simulink model "bd_par_auto2"  (Simulink 4.1.1)
settings: Solver=ode1  SolverMode=SingleTasking  StartTime=0.0  StopTime=max(cyc_mph(:,1))  FixedStep=1  MaxStep=1  RelTol=1e-3  AbsTol=1e-3
undefined symbols (not defined in the file): air_cp, amb_tmp, cs_charge_deplete_bool, cs_charge_trq, cs_electric_decel_spd, cs_electric_launch_spd_hi, cs_electric_launch_spd_lo, cs_hi_soc, cs_lo_soc, cs_min_trq_frac, cs_off_trq_frac, cyc_avg_time, cyc_cargo_mass, cyc_elevation_init, cyc_filter_bool, cyc_grade, cyc_mph, enable_stop, ess_cap_scale, ess_coulombic_eff, ess_init_soc, ess_max_ah_cap, ess_max_volts, ess_min_volts, ess_mod_airflow, ess_mod_cp, ess_mod_init_tmp, ess_module_mass, ess_module_num, ess_on, ess_res_scale_coef, ess_res_scale_fun, ess_set_tmp, ess_th_calc, ess_th_res_off, ess_th_res_on, ess_tmp, ess_voc, ex_calc, fc_ct_trq, fc_emis, fc_inertia, fc_map_spd, fc_max_trq, fc_on, fc_spd_scale, fc_trq_scale, fc_tstat, fd_inertia, fd_loss, fd_ratio, gb_dnshift_load, gb_dnshift_spd, gb_gears_num, gb_inertia, gb_num_init, gb_ratio, gb_shift_delay, gb_spd_scale, gb_trq_scale ... (+56)
libraries: lib_wheel2 x12, lib_accessory2 x3, lib_etc x2, lib_drive_cycle2 x1, lib_interactive x1, lib_drive_cycle x1, lib_exhaust x1, lib_fuel_converter3 x1
(part 1 of 18)
settings Model: LastModifiedBy=mokeefe  ModifiedComment=mokeefe -- Wed Apr 16 13:36:53 2003 -- Version 1.22  SaveTime=off  SaveOutput=off  LimitDataPoints=off  UnconnectedLineMsg=none  RTWTemplateMakefile=grt_vc.tmf  ExtModeTrigMode=oneshot  ExtModeArmWhenConnect=off
settings Model: ModifiedHistory=|
  | mokeefe -- Wed Apr 16 13:36:53 2003 -- Version 1.22
  | 
  | 
  | mokeefe -- Wed Apr 16 13:36:31 2003 -- Version 1.21
  | 
  | 
  | mokeefe -- Fri Aug 30 07:45:49 2002 -- Version 1.20
  | Changed the input to "mechanical accessory loads <acc>/Mechanical Accessory Loads V2 <acc>" masked parameter input blocks. In R13, the function "not" no longer returns double 1 or double 0 for true and false but instead returns type logical (boolean). Thus, I am now multiplying by double 1 which causes a type conversion to double yielding the desired effect.
  | 
  | 
  | abrooker -- Tue May 14 11:45:21 2002 -- Version 1.19
  | 
  | 
  | mokeefe -- Thu Apr 18 08:00:10 2002 -- Version 1.18
  | saving the model:
  | o "without the model browser open"
  | o with only top-level screen visible
  | o and with "fit to view" enabled

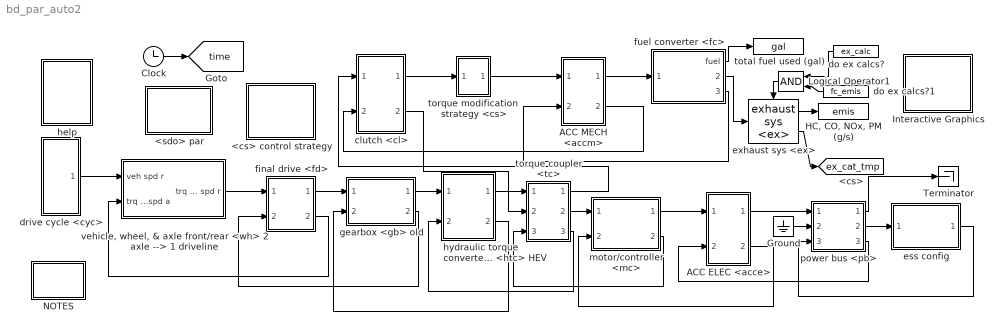
== system bd_par_auto2 ==
  <cs> control strategy : Subsystem
      settings: RTWFcnNameOpts=Auto  RTWFileNameOpts=Auto
      mask Display: image(imread('bdi_cs.jpg'))
  <sdo> par : Subsystem
      settings: RTWFcnNameOpts=Auto  RTWFileNameOpts=Auto
      mask Display: image(imread('bdi_sdo.jpg'))
  ACC ELEC <acce> : Subsystem  AncestorBlock=lib_accessory2/ACC ELEC <acce>  mask(Stand-Alone Electrical Accessory Mask){generalName='acce', logPick=Log, initFileName={}, modCell={}, imgFileName='bdi_acc_elec.bmp', DEBUG=OFF}
      mask prompts: generalName "General Name of this Component [char]"; logPick "Log Variables to Workspace?"; initFileName "Initialization File(s) [cell array of char]"; modCell "Modification Cell [2 column cell array of param and val]"; imgFileName "Icon image file name [char--evaluated]"
      mask init:
      | % initialization via m-file script
      | advSACompMaskInit;
      settings: RTWFcnNameOpts=Auto  RTWFileNameOpts=Auto
      mask StyleString: edit,popup(Don't Log|Log),edit,edit,edit,popup(ON|OFF)
      mask Display: image(imread(imgFileName))
  ACC MECH <accm> : Subsystem  AncestorBlock=lib_accessory2/ACC MECH <accm>  mask(Stand-Alone Mechanical Accessory Mask){generalName='accm', logPick=Log, initFileName={}, modCell={}, imgFileName='bdi_acc_pic.bmp', DEBUG=OFF}
      mask prompts: generalName "General Name of this Component [char]"; logPick "Log Variables to Workspace?"; initFileName "Initialization File(s) [cell array of char]"; modCell "Modification Cell [2 column cell array of param and val]"; imgFileName "Icon image file name [char--evaluated]"
      mask init:
      | % initialization via m-file script
      | advSACompMaskInit;
      settings: RTWFcnNameOpts=Auto  RTWFileNameOpts=Auto
      mask StyleString: edit,popup(Don't Log|Log),edit,edit,edit,popup(ON|OFF)
      mask Display: image(imread(imgFileName))
  Clock : Clock
      settings: DisplayTime=off  Decimation=10
  Ground : Ground
  "HC, CO, NOx, PM (g/s)" : ToWorkspace  VariableName=emis  SampleTime=0  SaveFormat=Array
  Interactive Graphics : Subsystem  BlockChoice=off
      settings: AttributesFormatString=%<BlockChoice>  TemplateBlock=lib_interactive/Interactive Graphics  MemberBlocks=off,on  RTWFcnNameOpts=Auto  RTWFileNameOpts=Auto
  Logical Operator1 : Logic  Orientation=left  Operator=AND  Inputs=2
  NOTES : Subsystem
      settings: RTWFcnNameOpts=Auto  RTWFileNameOpts=Auto
      mask Display: disp('Version &\nCopyright')
  Terminator : Terminator
  clutch <cl> : Subsystem  AncestorBlock=lib_transmission2/clutch <cl>  mask(Stand-Alone Clutch Mask){generalName='cl', logPick=Don't Log, initFileName={}, modCell={}, imgFileName='bdi_cl.jpg', slip_spd=vc_launch_spd, maxtrq=max(fc_max_trq)*fc_trq_scale, DEBUG=OFF}
      mask prompts: generalName "General Name of this Component [char--evaluated]"; logPick "Log Variables to Workspace?"; initFileName "Initialization File(s) [cell array of char]"; modCell "Modification Cell [2 column cell array of param and val]"; imgFileName "Icon image file name [char--evaluated]"; slip_spd "Input shaft speed when clutch slips (rad/s):"; maxtrq "Maximum torque clutch can transmit:"
      mask help: Clutch for use with ADVISOR 2
      mask init:
      | % initialization via m-file script
      | advSACompMaskInit;
      settings: RTWFcnNameOpts=Auto  RTWFileNameOpts=Auto
      mask Help:
      | First input is req'd clutch output torque and speed, muxed together.
      | Second input is clutch state, with 1 => disengaged, 2 => slipping, and 3=> engaged.
      | Third input is available clutch input torque and limited clutch input speed.
      | First output is req'd clutch input torque and speed, muxed together.
      | Second output is available clutch output torque and limited clutch output speed.
      | The logic implemented by this block is as follows:
      |           IF (clutch is disengaged) THEN (req'd input torque=0), (req'd input speed=req'd output speed (the engine control is responsible for computing correct engine spin-down speed)), (avail. output torque=0), (limited output speed=req'd output speed)
      |           IF (clutch is slipping) THEN (req'd input torque=req'd output torque), (req'd input speed=user-defined slip speed), (avail. output torque=avail. input torque), (limited output speed=req'd output speed)
      |           IF (clutch is engaged) THEN (req'd input torque=req'd output torque), (req'd input speed=req'd output speed), (avail. output torque=avail. input torque), (limited output speed=limited input speed)
      | 
      | The clutch will transmit no more than its maximum torque as driving or braking torque.
      mask StyleString: edit,popup(Don't Log|Log),edit,edit,edit,edit,edit,popup(ON|OFF)
      mask Display: image(imread(imgFileName))
  do ex calcs? : Constant  Orientation=left  Value=ex_calc
  do ex calcs?1 : Constant  Orientation=left  Value=fc_emis
  drive cycle <cyc> : Subsystem  AncestorBlock=lib_drive_cycle2/drive cycle <cyc>  mask(Stand-Alone Drive Cycle Mask){generalName='cyc', logPick=Log, initFileName={}, modCell={}, imgFileName='bdi_cyc.jpg', DEBUG=OFF, veh_mass=veh_mass}
      mask prompts: generalName "General Name of this Component [char]"; logPick "Log Variables to Workspace?"; initFileName "Initialization File(s) [cell array of char]"; modCell "Modification Cell [2 column cell array of param and val]"; imgFileName "Icon image file name [char--evaluated]"; veh_mass "Vehicle Mass (kg)"
      mask init:
      | % initialization via m-file script
      | advSACompMaskInit;
      settings: RTWFcnNameOpts=Auto  RTWFileNameOpts=Auto
      mask StyleString: edit,popup(Don't Log|Log),edit,edit,edit,popup(ON|OFF),edit
      mask Display: image(imread(imgFileName))
  ess config : Subsystem  BlockChoice=energy storage <ess>
      link override energy storage <ess>/controlTag: GotoTag=essControl
      link override energy storage <ess>/energy storage <ess>/Model/compute current/enhancedToWorkspace2/To Workspace: VariableName=ess_current  SampleTime=-1  SaveFormat=Array
      link override energy storage <ess>/energy storage <ess>/Model/enhancedToWorkspace/To Workspace: VariableName=ess_pwr_out_r  SampleTime=-1  SaveFormat=Array
      link override energy storage <ess>/energy storage <ess>/Model/enhancedToWorkspace1/To Workspace: VariableName=ess_pwr_loss_a  SampleTime=-1  SaveFormat=Array
      link override energy storage <ess>/energy storage <ess>/Model/enhancedToWorkspace2/To Workspace: VariableName=ess_mod_tmp  SampleTime=-1  SaveFormat=Array
      link override energy storage <ess>/energy storage <ess>/Model/enhancedToWorkspace3/To Workspace: VariableName=ess_air_tmp  SampleTime=-1  SaveFormat=Array
      link override energy storage <ess>/energy storage <ess>/Model/enhancedToWorkspace4/To Workspace: VariableName=ess_air_th_pwr  SampleTime=-1  SaveFormat=Array
      link override energy storage <ess>/energy storage <ess>/Model/enhancedToWorkspace5/To Workspace: VariableName=ess_pwr_out_a  SampleTime=-1  SaveFormat=Array
      link override energy storage <ess>/reqOutTag: GotoTag=essReqOut  TagVisibility=global
      link override energy storage <ess>/sensorsTag: GotoTag=essSensors  TagVisibility=global
      settings: AttributesFormatString=%<BlockChoice>  TemplateBlock=lib_energy_storage2/ess config  MemberBlocks="Ultracapacitor  System,energy storage <ess>,energy storage <ess> RC,energy storage <ess> nnet,energy storage <ess> Saber,energy storage <ess> fundamental model,energy storage <ess> optima fundamental model"  RTWFcnNameOpts=Auto  RTWFileNameOpts=Auto
  exhaust sys <ex> : lib_exhaust/exhaust sys <ex>
  final drive <fd> : Subsystem  AncestorBlock=lib_transmission2/final drive <fd>  mask(Stand-Alone Final Drive Mask){generalName='fd', logPick=Log, initFileName={}, modCell={}, imgFileName='bdi_fd.jpg', DEBUG=OFF}
      mask prompts: generalName "General Name of this Component [char]"; logPick "Log Variables to Workspace?"; initFileName "Initialization File(s) [cell array of char]"; modCell "Modification Cell [2 column cell array of param and val]"; imgFileName "Icon image file name [char--evaluated]"
      mask init:
      | % initialization via m-file script
      | advSACompMaskInit;
      settings: RTWFcnNameOpts=Auto  RTWFileNameOpts=Auto
      mask StyleString: edit,popup(Don't Log|Log),edit,edit,edit,popup(ON|OFF)
      mask Display: image(imread(imgFileName))
  fuel converter <fc> : Subsystem  AncestorBlock=lib_fuel_converter3/fuel converter <fc>  mask(Stand-Alone IC ENGINE Mask){generalName='fc', logPick=Log, initFileName={}, modCell={}, imgFileName='bdi_fc.jpg', DEBUG=OFF}
      mask prompts: generalName "General Name of this Component [char]"; logPick "Log Variables to Workspace?"; initFileName "Initialization File(s) [cell array of char]"; modCell "Modification Cell [2 column cell array of param and val]"; imgFileName "Icon image file name [char--evaluated]"
      mask init:
      | % initialization via m-file script
      | advSACompMaskInit;
      settings: RTWFcnNameOpts=Auto  RTWFileNameOpts=Auto
      mask StyleString: edit,popup(Don't Log|Log),edit,edit,edit,popup(ON|OFF)
      mask Display: image(imread(imgFileName))
  gearbox <gb> old : Subsystem  AncestorBlock=lib_transmission2/gearbox <gb> old  mask(Stand-Alone Gearbox Mask){generalName='gb', logPick=Log, initFileName={}, modCell={}, imgFileName='bdi_gb.jpg', DEBUG=OFF}
      mask prompts: generalName "General Name of this Component [char]"; logPick "Log Variables to Workspace?"; initFileName "Initialization File(s) [cell array of char]"; modCell "Modification Cell [2 column cell array of param and val]"; imgFileName "Icon image file name [char--evaluated]"
      mask init:
      | % initialization via m-file script
      | advSACompMaskInit;
      settings: RTWFcnNameOpts=Auto  RTWFileNameOpts=Auto
      mask StyleString: edit,popup(Don't Log|Log),edit,edit,edit,popup(ON|OFF)
      mask Display: image(imread(imgFileName))
  help : Subsystem
      settings: OpenFcn=web(['file:\\\' which('advisor_doc.htm')]);  RTWFcnNameOpts=Auto  RTWFileNameOpts=Auto
      mask Display: image(imread('doc_man.jpg'))
  hydraulic torque converter <htc> HEV : Subsystem  AncestorBlock=|  mask(Stand-Alone HTC Mask){generalName='htc', logPick=Log, initFileName={}, modCell={}, imgFileName='bdi_htc.jpg', DEBUG=OFF}
      | lib_transmission2/hydraulic
      | torque
      | converter <htc>
      | HEV
      mask prompts: generalName "General Name of this Component [char]"; logPick "Log Variables to Workspace?"; initFileName "Initialization File(s) [cell array of char]"; modCell "Modification Cell [2 column cell array of param and val]"; imgFileName "Icon image file name [char--evaluated]"
      mask init:
      | % initialization via m-file script
      | advSACompMaskInit;
      settings: RTWFcnNameOpts=Auto  RTWFileNameOpts=Auto
      mask StyleString: edit,popup(Don't Log|Log),edit,edit,edit,popup(ON|OFF)
      mask Display: image(imread(imgFileName))
  motor/controller <mc> : Subsystem  AncestorBlock=lib_electric_machine2/motor//controller <mc>  mask(Stand-Alone Motor/Controller Mask){generalName='mc', logPick=Log, initFileName={}, modCell={}, imgFileName='bdi_mc.jpg', DEBUG=OFF}
      mask prompts: generalName "General Name of this Component [char]"; logPick "Log Variables to Workspace?"; initFileName "Initialization File(s) [cell array of char]"; modCell "Modification Cell [2 column cell array of param and val]"; imgFileName "Icon image file name [char--evaluated]"
      mask init:
      | % initialization via m-file script
      | advSACompMaskInit;
      settings: RTWFcnNameOpts=Auto  RTWFileNameOpts=Auto
      mask StyleString: edit,popup(Don't Log|Log),edit,edit,edit,popup(ON|OFF)
      mask Display: image(imread(imgFileName))
  power bus <pb> : Subsystem  AncestorBlock=lib_power_bus2/power bus <pb>  mask(Stand-Alone Power Bus Mask){generalName='pb', logPick=Log, initFileName={}, modCell={}, imgFileName='bdi_pb.jpg', DEBUG=OFF}
      mask prompts: generalName "General Name of this Component [char]"; logPick "Log Variables to Workspace?"; initFileName "Initialization File(s) [cell array of char]"; modCell "Modification Cell [2 column cell array of param and val]"; imgFileName "Icon image file name [char--evaluated]"
      mask init:
      | % initialization via m-file script
      | advSACompMaskInit;
      settings: RTWFcnNameOpts=Auto  RTWFileNameOpts=Auto
      mask StyleString: edit,popup(Don't Log|Log),edit,edit,edit,popup(ON|OFF)
      mask Display: image(imread(imgFileName))
  torque coupler <tc> : Subsystem  AncestorBlock=lib_transmission2/torque coupler <tc>  mask(Stand-Alone Torque Coupler Mask){generalName='tc', logPick=Don't Log, initFileName={}, modCell={}, imgFileName='bdi_tc.jpg', DEBUG=OFF}
      mask prompts: generalName "General Name of this Component [char--evaluated]"; logPick "Log Variables to Workspace?"; initFileName "Initialization File(s) [cell array of char]"; modCell "Modification Cell [2 column cell array of param and val]"; imgFileName "Icon image file name [char--evaluated]"
      mask init:
      | % initialization via m-file script
      | advSACompMaskInit;
      settings: RTWFcnNameOpts=Auto  RTWFileNameOpts=Auto
      mask StyleString: edit,popup(Don't Log|Log),edit,edit,edit,popup(ON|OFF)
      mask Display: image(imread(imgFileName))
  torque modification  strategy <cs> : Subsystem  mask(Stand-Alone Torque Modification Strategy Mask){generalName='tm', logPick=Log, initFileName={}, modCell={}, imgFileName='bdi_hybrid_cntrl.jpg', DEBUG=OFF}
      mask prompts: generalName "General Name of this Component [char]"; logPick "Log Variables to Workspace?"; initFileName "Initialization File(s) [cell array of char]"; modCell "Modification Cell [2 column cell array of param and val]"; imgFileName "Icon image file name [char--evaluated]"
      mask init:
      | % initialization via m-file script
      | advSACompMaskInit;
      settings: RTWFcnNameOpts=Auto  RTWFileNameOpts=Auto
      mask StyleString: edit,popup(Don't Log|Log),edit,edit,edit,popup(ON|OFF)
      mask Display: image(imread(imgFileName))
  total fuel used (gal) : ToWorkspace  VariableName=gal  SampleTime=0  SaveFormat=Array
  "vehicle, wheel, & axle front/rear <wh> 2 axle --> 1 driveline" : Subsystem  AncestorBlock=|  mask(Stand-Alone Vehicle, Wheel, & Axle Mask){generalName='veh', generalName01='wh', logPick=Log, initFileName={}, modCell={}, imgFileName='bdi_wh&veh.jpg', DEBUG=OFF}
      | lib_wheel2/vehicle, wheel, & axle
      | front//rear <wh>
      | 2 axle --> 1 driveline
      mask prompts: generalName "General Name of Vehicle Component [char]"; generalName01 "General Name of Wheel Component [char]"; logPick "Log Variables to Workspace?"; initFileName "Initialization File(s) for VEH and WH [cell array of char]"; modCell "Modification Cell [2 column cell array of param and val]"; imgFileName "Icon image file name [char--evaluated]"
      mask init:
      | % initialization via m-file script
      | advSACompMaskInit;
      settings: RTWFcnNameOpts=Auto  RTWFileNameOpts=Auto
      mask StyleString: edit,edit,popup(Don't Log|Log),edit,edit,edit,popup(ON|OFF)
      mask Display: image(imread(imgFileName))
  tag scope: ex_cat_tmp=global, time=global
  wires:
  "vehicle, wheel, & axle front/rear <wh> 2 axle --> 1 driveline"/1(trq & spd r) -> final drive <fd>/1("torque and speed req'd at output side of final drive (Nm), (rad/s)")
  final drive <fd>/2("torque and speed avail. at output side of final drive (Nm), (rad/s)") -> "vehicle, wheel, & axle front/rear <wh> 2 axle --> 1 driveline"/2(trq & spd a)
  final drive <fd>/1("torque and speed req'd at input side of final drive (Nm), (rad/s)") -> gearbox <gb> old/1("torque and speed req'd at output side of gearbox (Nm), (rad/s)")
  drive cycle <cyc>/1(req'd vehicle speed (m/s)) -> "vehicle, wheel, & axle front/rear <wh> 2 axle --> 1 driveline"/1(veh spd r)
  clutch <cl>/1(T & w input request) -> torque modification  strategy <cs>/1("original torque and speed req'd (Nm), (rad/s)")
  fuel converter <fc>/2(engine out emissions) -> exhaust sys <ex>/1
  do ex calcs?/1 -> Logical Operator1/1
  fuel converter <fc>/1(fuel) -> total fuel used (gal)/1
  exhaust sys <ex>/1 -> "HC, CO, NOx, PM (g/s)"/1
  Logical Operator1/1 -> exhaust sys <ex>/Enable
  do ex calcs?1/1 -> Logical Operator1/2
  Clock/1 -> [time]
  gearbox <gb> old/2("torque and speed avail. at output side of gearbox (Nm), (rad/s)") -> final drive <fd>/2("torque and speed avail. at input side of final drive (Nm), (rad/s)")
  clutch <cl>/2(T & w output achieved) -> torque coupler <tc>/2("torque and speed avail. at main input (Nm), (rad/s)")
  torque coupler <tc>/1("torque and speed req'd at main input to torque coupler (Nm), (rad/s)") -> clutch <cl>/1(T & w output requested)
  motor/controller <mc>/2("trq and spd out achieved ") -> torque coupler <tc>/3("torque and speed avail. at motor input to tc (Nm), (rad/s)")
  Ground/1 -> power bus <pb>/2(power available from source one (W))
  power bus <pb>/2(power req'd from source two (W)) -> ess config/1(power req'd into bus (W))
  power bus <pb>/1(power req'd from source one (W)) -> Terminator/1
  ess config/1(power available to bus (W)) -> power bus <pb>/3(power available from source two (W))
  torque coupler <tc>/2("torque and speed req'd at motor input to torque coupler (Nm), (rad/s)") -> motor/controller <mc>/1(trq and spd out requested)
  gearbox <gb> old/1("torque and speed req'd at input side of gearbox (Nm), (rad/s)") -> hydraulic torque converter <htc> HEV/1(T & w output requested)
  hydraulic torque converter <htc> HEV/1(T & w input requested) -> torque coupler <tc>/1("torque and speed req'd at output side of torque coupler (Nm), (rad/s)")
  hydraulic torque converter <htc> HEV/2(T & w output available) -> gearbox <gb> old/2("torque and speed avail. at input side of gearbox (Nm), (rad/s)")
  torque coupler <tc>/3("torque and speed avail. at output side of torque coupler (Nm), (rad/s)") -> hydraulic torque converter <htc> HEV/2(T & w input available)
  exhaust sys <ex>/2 -> [ex_cat_tmp]
  motor/controller <mc>/1(electric power in  requested) -> ACC ELEC <acce>/1(elec pwr out r (W))
  ACC ELEC <acce>/1(elec pwr in r (W)) -> power bus <pb>/1(req'd power output (W))
  power bus <pb>/3(output power  available at bus) -> ACC ELEC <acce>/2(elec pwr in a (W))
  ACC ELEC <acce>/2(elec pwr out a (W)) -> motor/controller <mc>/2(electric power in achieved)
  torque modification  strategy <cs>/1("modified torque and speed req'd (Nm), (rad/s)") -> ACC MECH <accm>/1(trq and spd out requested)
  ACC MECH <accm>/1(trq and spd in  requested) -> fuel converter <fc>/1(trq and spd out requested)
  fuel converter <fc>/3(trq and spd out achieved) -> ACC MECH <accm>/2(trq and spd in achieved)
  ACC MECH <accm>/2("trq and spd out achieved ") -> clutch <cl>/2(T & w input achieved)

== system bd_par_auto2/<cs> control strategy ==
  Automatic Transmission  Control : Subsystem
      settings: RTWFcnNameOpts=Auto  RTWFileNameOpts=Auto
  Clutch Control : Subsystem
      settings: RTWFcnNameOpts=Auto  RTWFileNameOpts=Auto
  Drive Cycle : Subsystem
      settings: RTWFcnNameOpts=Auto  RTWFileNameOpts=Auto
  Electrical Accessories : Subsystem
      settings: RTWFcnNameOpts=Auto  RTWFileNameOpts=Auto
  Fuel Converter Control parallel hybrid  ic engine : Subsystem
      settings: RTWFcnNameOpts=Auto  RTWFileNameOpts=Auto
  Hybrid  Engine Torque Modification Strategy : Subsystem
      settings: RTWFcnNameOpts=Auto  RTWFileNameOpts=Auto
      mask Display: image(imread('bdi_hybrid_cntrl.jpg'))
  Mechanical Accessories : Subsystem
      settings: RTWFcnNameOpts=Auto  RTWFileNameOpts=Auto
  Motor Controller : Subsystem
      settings: RTWFcnNameOpts=Auto  RTWFileNameOpts=Auto
  Power Bus : Subsystem
      settings: RTWFcnNameOpts=Auto  RTWFileNameOpts=Auto
  Wheel Control : Subsystem
      settings: RTWFcnNameOpts=Auto  RTWFileNameOpts=Auto

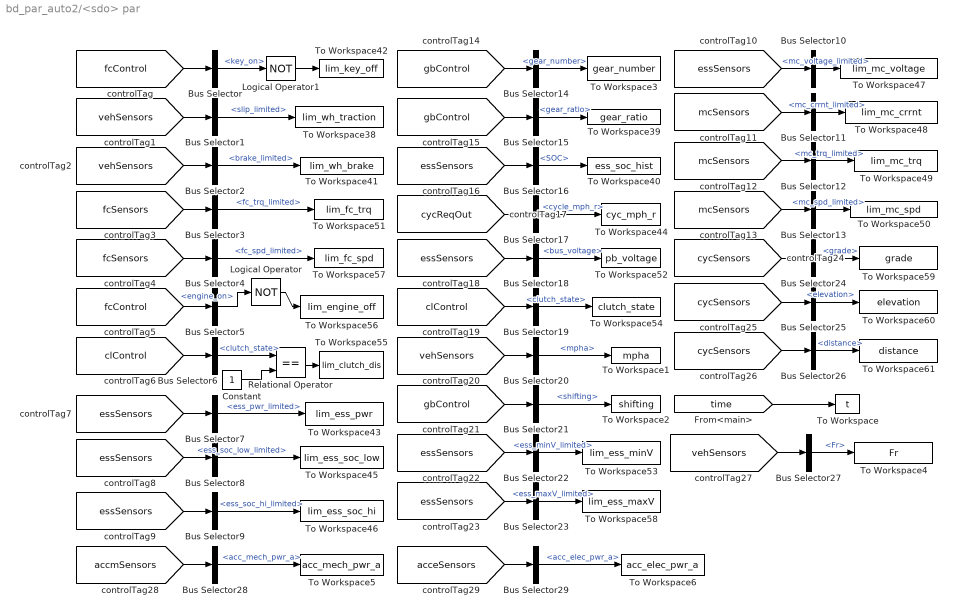
== system bd_par_auto2/<sdo> par ==
  Bus Selector : BusSelector  OutputSignals=key_on  MuxedOutput=off
  Bus Selector1 : BusSelector  OutputSignals=slip_limited  MuxedOutput=off
  Bus Selector10 : BusSelector  OutputSignals=mc_voltage_limited  MuxedOutput=off
  Bus Selector11 : BusSelector  OutputSignals=mc_crrnt_limited  MuxedOutput=off
  Bus Selector12 : BusSelector  OutputSignals=mc_trq_limited  MuxedOutput=off
  Bus Selector13 : BusSelector  OutputSignals=mc_spd_limited  MuxedOutput=off
  Bus Selector14 : BusSelector  OutputSignals=gear_number  MuxedOutput=off
  Bus Selector15 : BusSelector  OutputSignals=gear_ratio  MuxedOutput=off
  Bus Selector16 : BusSelector  OutputSignals=SOC  MuxedOutput=off
  Bus Selector17 : BusSelector  OutputSignals=cycle_mph_r  MuxedOutput=off
  Bus Selector18 : BusSelector  OutputSignals=bus_voltage  MuxedOutput=off
  Bus Selector19 : BusSelector  OutputSignals=clutch_state  MuxedOutput=off
  Bus Selector2 : BusSelector  OutputSignals=brake_limited  MuxedOutput=off
  Bus Selector20 : BusSelector  OutputSignals=mpha  MuxedOutput=off
  Bus Selector21 : BusSelector  OutputSignals=shifting  MuxedOutput=off
  Bus Selector22 : BusSelector  OutputSignals=ess_minV_limited  MuxedOutput=off
  Bus Selector23 : BusSelector  OutputSignals=ess_maxV_limited  MuxedOutput=off
  Bus Selector24 : BusSelector  OutputSignals=grade  MuxedOutput=off
  Bus Selector25 : BusSelector  OutputSignals=elevation  MuxedOutput=off
  Bus Selector26 : BusSelector  OutputSignals=distance  MuxedOutput=off
  Bus Selector27 : BusSelector  OutputSignals=Fr  MuxedOutput=off
  Bus Selector28 : BusSelector  OutputSignals=acc_mech_pwr_a  MuxedOutput=off
  Bus Selector29 : BusSelector  OutputSignals=acc_elec_pwr_a  MuxedOutput=off
  Bus Selector3 : BusSelector  OutputSignals=fc_trq_limited  MuxedOutput=off
  Bus Selector4 : BusSelector  OutputSignals=fc_spd_limited  MuxedOutput=off
  Bus Selector5 : BusSelector  OutputSignals=engine_on  MuxedOutput=off
  Bus Selector6 : BusSelector  OutputSignals=clutch_state  MuxedOutput=off
  Bus Selector7 : BusSelector  OutputSignals=ess_pwr_limited  MuxedOutput=off
  Bus Selector8 : BusSelector  OutputSignals=ess_soc_low_limited  MuxedOutput=off
  Bus Selector9 : BusSelector  OutputSignals=ess_soc_hi_limited  MuxedOutput=off
  Constant : Constant  Value=1
  Logical Operator : Logic  Operator=NOT  Inputs=1
  Logical Operator1 : Logic  Operator=NOT  Inputs=1
  Relational Operator : RelationalOperator  Operator===
  To Workspace : ToWorkspace  VariableName=t  SampleTime=0  SaveFormat=Array
  To Workspace1 : ToWorkspace  VariableName=mpha  SampleTime=-1  SaveFormat=Array
  To Workspace2 : ToWorkspace  VariableName=shifting  SampleTime=-1  SaveFormat=Array
  To Workspace3 : ToWorkspace  VariableName=gear_number  SampleTime=-1  SaveFormat=Array
  To Workspace38 : ToWorkspace  VariableName=lim_wh_traction  SampleTime=-1  SaveFormat=Array
  To Workspace39 : ToWorkspace  VariableName=gear_ratio  SampleTime=-1  SaveFormat=Array
  To Workspace4 : ToWorkspace  VariableName=Fr  SampleTime=-1  SaveFormat=Array
  To Workspace40 : ToWorkspace  VariableName=ess_soc_hist  SampleTime=-1  SaveFormat=Array
  To Workspace41 : ToWorkspace  VariableName=lim_wh_brake  SampleTime=-1  SaveFormat=Array
  To Workspace42 : ToWorkspace  VariableName=lim_key_off  SampleTime=-1  SaveFormat=Array
  To Workspace43 : ToWorkspace  VariableName=lim_ess_pwr  SampleTime=-1  SaveFormat=Array
  To Workspace44 : ToWorkspace  VariableName=cyc_mph_r  SampleTime=-1  SaveFormat=Array
  To Workspace45 : ToWorkspace  VariableName=lim_ess_soc_low  SampleTime=-1  SaveFormat=Array
  To Workspace46 : ToWorkspace  VariableName=lim_ess_soc_hi  SampleTime=-1  SaveFormat=Array
  To Workspace47 : ToWorkspace  VariableName=lim_mc_voltage  SampleTime=-1  SaveFormat=Array
  To Workspace48 : ToWorkspace  VariableName=lim_mc_crrnt  SampleTime=-1  SaveFormat=Array
  To Workspace49 : ToWorkspace  VariableName=lim_mc_trq  SampleTime=-1  SaveFormat=Array
  To Workspace5 : ToWorkspace  VariableName=acc_mech_pwr_a  SampleTime=-1  SaveFormat=Array
  To Workspace50 : ToWorkspace  VariableName=lim_mc_spd  SampleTime=-1  SaveFormat=Array
  To Workspace51 : ToWorkspace  VariableName=lim_fc_trq  SampleTime=-1  SaveFormat=Array
  To Workspace52 : ToWorkspace  VariableName=pb_voltage  SampleTime=-1  SaveFormat=Array
  To Workspace53 : ToWorkspace  VariableName=lim_ess_minV  SampleTime=-1  SaveFormat=Array
  To Workspace54 : ToWorkspace  VariableName=clutch_state  SampleTime=-1  SaveFormat=Array
  To Workspace55 : ToWorkspace  VariableName=lim_clutch_dis  SampleTime=-1  SaveFormat=Array
  To Workspace56 : ToWorkspace  VariableName=lim_engine_off  SampleTime=-1  SaveFormat=Array
  To Workspace57 : ToWorkspace  VariableName=lim_fc_spd  SampleTime=-1  SaveFormat=Array
  To Workspace58 : ToWorkspace  VariableName=lim_ess_maxV  SampleTime=-1  SaveFormat=Array
  To Workspace59 : ToWorkspace  VariableName=grade  SampleTime=-1  SaveFormat=Array
  To Workspace6 : ToWorkspace  VariableName=acc_elec_pwr_a  SampleTime=-1  SaveFormat=Array
  To Workspace60 : ToWorkspace  VariableName=elevation  SampleTime=-1  SaveFormat=Array
  To Workspace61 : ToWorkspace  VariableName=distance  SampleTime=-1  SaveFormat=Array
  wires:
  [time] -> To Workspace/1
  Logical Operator/1 -> To Workspace56/1
  Bus Selector1/1 -> To Workspace38/1  "<slip_limited>"
  Logical Operator1/1 -> To Workspace42/1
  [fcControl] -> Bus Selector/1
  Bus Selector/1 -> Logical Operator1/1  "<key_on>"
  [vehSensors] -> Bus Selector1/1
  Bus Selector2/1 -> To Workspace41/1  "<brake_limited>"
  [vehSensors] -> Bus Selector2/1
  [fcSensors] -> Bus Selector3/1
  Bus Selector3/1 -> To Workspace51/1  "<fc_trq_limited>"
  [fcSensors] -> Bus Selector4/1
  Bus Selector4/1 -> To Workspace57/1  "<fc_spd_limited>"
  [fcControl] -> Bus Selector5/1
  Bus Selector5/1 -> Logical Operator/1  "<engine_on>"
  [clControl] -> Bus Selector6/1
  Relational Operator/1 -> To Workspace55/1
  Constant/1 -> Relational Operator/2
  Bus Selector6/1 -> Relational Operator/1  "<clutch_state>"
  [essSensors] -> Bus Selector7/1
  Bus Selector7/1 -> To Workspace43/1  "<ess_pwr_limited>"
  [essSensors] -> Bus Selector8/1
  Bus Selector8/1 -> To Workspace45/1  "<ess_soc_low_limited>"
  [essSensors] -> Bus Selector9/1
  Bus Selector9/1 -> To Workspace46/1  "<ess_soc_hi_limited>"
  [essSensors] -> Bus Selector10/1
  Bus Selector10/1 -> To Workspace47/1  "<mc_voltage_limited>"
  [mcSensors] -> Bus Selector11/1
  Bus Selector11/1 -> To Workspace48/1  "<mc_crrnt_limited>"
  [mcSensors] -> Bus Selector12/1
  Bus Selector12/1 -> To Workspace49/1  "<mc_trq_limited>"
  [mcSensors] -> Bus Selector13/1
  Bus Selector13/1 -> To Workspace50/1  "<mc_spd_limited>"
  [gbControl] -> Bus Selector14/1
  Bus Selector14/1 -> To Workspace3/1  "<gear_number>"
  [gbControl] -> Bus Selector15/1
  Bus Selector15/1 -> To Workspace39/1  "<gear_ratio>"
  [essSensors] -> Bus Selector16/1
  Bus Selector16/1 -> To Workspace40/1  "<SOC>"
  [cycReqOut] -> Bus Selector17/1
  Bus Selector17/1 -> To Workspace44/1  "<cycle_mph_r>"
  [essSensors] -> Bus Selector18/1
  Bus Selector18/1 -> To Workspace52/1  "<bus_voltage>"
  [clControl] -> Bus Selector19/1
  Bus Selector19/1 -> To Workspace54/1  "<clutch_state>"
  [vehSensors] -> Bus Selector20/1
  Bus Selector20/1 -> To Workspace1/1  "<mpha>"
  [gbControl] -> Bus Selector21/1
  Bus Selector21/1 -> To Workspace2/1  "<shifting>"
  [essSensors] -> Bus Selector22/1
  Bus Selector22/1 -> To Workspace53/1  "<ess_minV_limited>"
  [essSensors] -> Bus Selector23/1
  Bus Selector23/1 -> To Workspace58/1  "<ess_maxV_limited>"
  [cycSensors] -> Bus Selector24/1
  Bus Selector24/1 -> To Workspace59/1  "<grade>"
  [cycSensors] -> Bus Selector25/1
  Bus Selector25/1 -> To Workspace60/1  "<elevation>"
  [cycSensors] -> Bus Selector26/1
  Bus Selector26/1 -> To Workspace61/1  "<distance>"
  [vehSensors] -> Bus Selector27/1
  Bus Selector27/1 -> To Workspace4/1  "<Fr>"
  [accmSensors] -> Bus Selector28/1
  Bus Selector28/1 -> To Workspace5/1  "<acc_mech_pwr_a>"
  [acceSensors] -> Bus Selector29/1
  Bus Selector29/1 -> To Workspace6/1  "<acc_elec_pwr_a>"

== system bd_par_auto2/ACC ELEC <acce> ==
  note: ELECTRICAL ACCESSORY
      | Interface
  elec pwr out r (W) : Inport  Port=1  LatchInput=off
  elec pwr in a (W) : Inport  Port=2  LatchInput=off
  ACC ELEC model and interface : lib_accessory2/ACC ELEC <acce>/ACC ELEC model and interface
      link override electrical accessory model/backward model/electrical accessories (W): BlockChoice=Electrical Accessories: Time Variable
  elec pwr in r (W) : Outport  Port=1
  elec pwr out a (W) : Outport  Port=2
  tag scope: acceReqOut=global, acceSensors=global
  wires:
  [acceControl] -> ACC ELEC model and interface/3
  elec pwr out r (W)/1 -> ACC ELEC model and interface/1
  elec pwr in a (W)/1 -> ACC ELEC model and interface/2
  ACC ELEC model and interface/1 -> [acceReqOut]
  ACC ELEC model and interface/2 -> elec pwr in r (W)/1
  ACC ELEC model and interface/3 -> elec pwr out a (W)/1
  ACC ELEC model and interface/4 -> [acceSensors]

== system bd_par_auto2/ACC MECH <accm> ==
  note: MECHANICAL ACCESSORY
      | Interface
  trq and spd out requested : Inport  Port=1  LatchInput=off
  trq and spd in achieved : Inport  Port=2  LatchInput=off
  mechanical accessory model and interface : Subsystem  AncestorBlock=lib_accessory2/ACC MECH <accm>/mechanical accessory model and interface
      settings: RTWFcnNameOpts=Auto  RTWFileNameOpts=Auto
  trq and spd in  requested : Outport  Port=1
  "trq and spd out achieved " : Outport  Port=2
  tag scope: accmReqOut=global, accmSensors=global
  wires:
  mechanical accessory model and interface/4(sensors) -> [accmSensors]
  [accmControl] -> mechanical accessory model and interface/3(control)
  mechanical accessory model and interface/1(Out Request) -> [accmReqOut]
  mechanical accessory model and interface/2(T,w in request) -> trq and spd in  requested/1
  trq and spd out requested/1 -> mechanical accessory model and interface/1("T, w out requested")
  trq and spd in achieved/1 -> mechanical accessory model and interface/2("T, w in achieved")
  mechanical accessory model and interface/3("T, w out achieved") -> "trq and spd out achieved "/1

== system bd_par_auto2/Interactive Graphics ==
  off : lib_interactive/off  Tag=Altia_off  Orientation=up

== system bd_par_auto2/NOTES ==
  note: ADVISOR software developed at NREL.  Copyright 1998 Midwest Research Institute.  All rights reserved.
      | Notice: These data were produced by the Midwest Research Institute (MRI) under Contract No. DE-AC98GO10337
      |      with the Department of Energy (DOE).  For a five-year period from November 6, 1998, the Government is granted for
      | itself and others acting on its behalf a nonexclusive, paid-up, irrevocable worldwide license in this data to reproduce,
      |  prepare derivative works, and perform publicly and display publicly, by or on behalf of the Government.  There is
      | provision for the possible extension of the term of this license.  Subsequent to that period or any extension granted,
      |  the Government is granted for itself and others acting on its behalf a nonexclusive, paid-up, irrevocable worldwide
  note: license in this data to reproduce, prepare derivative works, distribute copies to the public, perform publicly and display
      | publicly, and to permit others to do so.  The specific term of the license can be identified by inquiry made to the MRI
      | or DOE. Neither the United States nor the DOE, nor any of their employees, make any warranty, express or implied, or
      | assumes any legal liability or responsibility for the accuracy, completeness, or usefulness of any data, apparatus,
      | product, or process disclosed, or represents that its use would not infringe privately owned rights.
  NOTES : Subsystem
      settings: OpenFcn=advisor_ver  RTWFcnNameOpts=Auto  RTWFileNameOpts=Auto
      mask Display: disp('Double-click here or enter ''advisor_ver'' at the Matlab\ncommand line for ADVISOR version')

== system bd_par_auto2/clutch <cl> ==
  note: Clutch
      | Interface
  T & w output requested : Inport  Port=1  LatchInput=off
  T & w input achieved : Inport  Port=2  LatchInput=off
  clutch model and interface : Subsystem
      settings: RTWFcnNameOpts=Auto  RTWFileNameOpts=Auto
  T & w input request : Outport  Port=1
  T & w output achieved : Outport  Port=2
  tag scope: clReqOut=global, clSensors=global
  wires:
  [clControl] -> clutch model and interface/3(control)
  clutch model and interface/1(required out) -> [clReqOut]
  clutch model and interface/4(sensors) -> [clSensors]
  clutch model and interface/3(Out2) -> T & w output achieved/1
  T & w input achieved/1 -> clutch model and interface/2(T & w input achieved)
  clutch model and interface/2(Out1) -> T & w input request/1
  T & w output requested/1 -> clutch model and interface/1(T & w output requested)

== system bd_par_auto2/drive cycle <cyc> ==
  note: DRIVE CYCLE
  drive cycle model and interface : Subsystem
      settings: RTWFcnNameOpts=Auto  RTWFileNameOpts=Auto
  req'd vehicle speed (m/s) : Outport  Port=1  InitialOutput=0
  tag scope: cycReqOut=global, cycSensors=global
  wires:
  drive cycle model and interface/3(sensors) -> [cycSensors]
  drive cycle model and interface/1(req'd lookups) -> [cycReqOut]
  [cycControl] -> drive cycle model and interface/1(control)
  drive cycle model and interface/2(req'd vehicle speed (m/s)) -> req'd vehicle speed (m/s)/1

== system bd_par_auto2/ess config ==
  power req'd into bus (W) : Inport  Port=1  LatchInput=off
  energy storage <ess> : Subsystem  AncestorBlock=lib_energy_storage2/energy storage <ess>  mask(Stand-Alone Energy Storage System Mask){generalName='ess', logPick=Log Variable, initFileName={}, modCell={}, imgFileName='bdi_ess.jpg', DEBUG=OFF}
      mask prompts: generalName "General Name of this Component [char]"; logPick "Log Variables to Workspace?"; initFileName "Initialization File(s) [cell array of char]"; modCell "Modification Cell [2 column cell array of param and val]"; imgFileName "Icon image file name [char--evaluated]"
      mask init:
      | % initialization via m-file script
      | advSACompMaskInit;
      settings: RTWFcnNameOpts=Auto  RTWFileNameOpts=Auto
      mask StyleString: edit,popup(Don't Log|Log Variable),edit,edit,edit,popup(ON|OFF)
      mask Display: image(imread(imgFileName))
  power available to bus (W) : Outport  Port=1
  wires:
  power req'd into bus (W)/1 -> energy storage <ess>/1(power req'd into bus (W))
  energy storage <ess>/1(power available to bus (W)) -> power available to bus (W)/1

== system bd_par_auto2/final drive <fd> ==
  "torque and speed req'd at output side of final drive (Nm), (rad/s)" : Inport  Port=1  LatchInput=off
  "torque and speed avail. at input side of final drive (Nm), (rad/s)" : Inport  Port=2  LatchInput=off
  Block NOTES : Subsystem
      settings: RTWFcnNameOpts=Auto  RTWFileNameOpts=Auto
      mask Display: disp('Block\nNOTES')
  help : Subsystem
      settings: OpenFcn=web(['file:\\\' which('wheel_axle.htm')]);  RTWFcnNameOpts=Auto  RTWFileNameOpts=Auto
      mask Display: image(imread('doc_man.jpg'))
  model&interface : Subsystem
      settings: RTWFcnNameOpts=Auto  RTWFileNameOpts=Auto
  "torque and speed req'd at input side of final drive (Nm), (rad/s)" : Outport  Port=1  InitialOutput=0
  "torque and speed avail. at output side of final drive (Nm), (rad/s)" : Outport  Port=2  InitialOutput=0
  tag scope: fdReqOut=global, fdSensors=global
  wires:
  model&interface/3(T & w output achieved) -> "torque and speed avail. at output side of final drive (Nm), (rad/s)"/1
  model&interface/2(T & w input request) -> "torque and speed req'd at input side of final drive (Nm), (rad/s)"/1
  "torque and speed avail. at input side of final drive (Nm), (rad/s)"/1 -> model&interface/2(T & w input achieved)
  "torque and speed req'd at output side of final drive (Nm), (rad/s)"/1 -> model&interface/1(T & w output request)
  model&interface/4(sensors) -> [fdSensors]
  [fdControl] -> model&interface/3(control)
  model&interface/1(out request) -> [fdReqOut]

== system bd_par_auto2/fuel converter <fc> ==
  note: Internal Combustion Engine
  trq and spd out requested : Inport  Port=1  LatchInput=off
  Block NOTES : Subsystem
      settings: RTWFcnNameOpts=Auto  RTWFileNameOpts=Auto
      mask Display: disp('Block\nNOTES')
  IC Engine Model  &  Interface : Subsystem
      settings: RTWFcnNameOpts=Auto  RTWFileNameOpts=Auto
  help : Subsystem
      settings: OpenFcn=web(['file:\\\' which('fuel_converter.htm')]);  RTWFcnNameOpts=Auto  RTWFileNameOpts=Auto
      mask Display: image(imread('doc_man.jpg'))
  fuel : Outport  Port=1
  engine out emissions : Outport  Port=2
  trq and spd out achieved : Outport  Port=3
  tag scope: fcReqOut=global, fcSensors=global
  wires:
  IC Engine Model  &  Interface/1(req out) -> [fcReqOut]
  IC Engine Model  &  Interface/2(fuel) -> fuel/1
  IC Engine Model  &  Interface/3(engine out emissions) -> engine out emissions/1
  IC Engine Model  &  Interface/4(trq and spd out achieved) -> trq and spd out achieved/1
  IC Engine Model  &  Interface/5(sensors) -> [fcSensors]
  [fcControl] -> IC Engine Model  &  Interface/2(control)
  trq and spd out requested/1 -> IC Engine Model  &  Interface/1(trq and spd out requested)

== system bd_par_auto2/gearbox <gb> old ==
  note: Gearbox
  "torque and speed req'd at output side of gearbox (Nm), (rad/s)" : Inport  Port=1  LatchInput=off
  "torque and speed avail. at input side of gearbox (Nm), (rad/s)" : Inport  Port=2  LatchInput=off
  Block NOTES : Subsystem
      settings: RTWFcnNameOpts=Auto  RTWFileNameOpts=Auto
      mask Display: disp('Block\nNOTES')
  gearbox model & interface : Subsystem
      settings: RTWFcnNameOpts=Auto  RTWFileNameOpts=Auto
  help : Subsystem
      settings: OpenFcn=web(['file:\\\' which('gearbox.htm')]);  RTWFcnNameOpts=Auto  RTWFileNameOpts=Auto
      mask Display: image(imread('doc_man.jpg'))
  "torque and speed req'd at input side of gearbox (Nm), (rad/s)" : Outport  Port=1  InitialOutput=0
  "torque and speed avail. at output side of gearbox (Nm), (rad/s)" : Outport  Port=2  InitialOutput=0
  tag scope: gbReqOut=global, gbSensors=global
  wires:
  gearbox model & interface/4(sensors) -> [gbSensors]
  [gbControl] -> gearbox model & interface/3(controls)
  gearbox model & interface/3(trq and spd output achieved) -> "torque and speed avail. at output side of gearbox (Nm), (rad/s)"/1
  "torque and speed avail. at input side of gearbox (Nm), (rad/s)"/1 -> gearbox model & interface/2(trq and spd input achieved)
  "torque and speed req'd at output side of gearbox (Nm), (rad/s)"/1 -> gearbox model & interface/1(trq and spd output request)
  gearbox model & interface/2(trq and spd input request) -> "torque and speed req'd at input side of gearbox (Nm), (rad/s)"/1
  gearbox model & interface/1(requested output) -> [gbReqOut]

== system bd_par_auto2/help ==

== system bd_par_auto2/hydraulic torque converter <htc> HEV ==
  note: Hydraulic Torque Converter
  T & w output requested : Inport  Port=1  LatchInput=off
  T & w input available : Inport  Port=2  LatchInput=off
  HTC for parallel HEV and Interface : Subsystem
      settings: RTWFcnNameOpts=Auto  RTWFileNameOpts=Auto
  T & w input requested : Outport  Port=1  InitialOutput=0
  T & w output available : Outport  Port=2  InitialOutput=0
  tag scope: htcReqOut=global, htcSensors=global
  wires:
  [htcControl] -> HTC for parallel HEV and Interface/3(control)
  T & w input available/1 -> HTC for parallel HEV and Interface/2(trq and spd input achieved)
  T & w output requested/1 -> HTC for parallel HEV and Interface/1(trq and spd output request)
  HTC for parallel HEV and Interface/3(trq and spd output achieved) -> T & w output available/1
  HTC for parallel HEV and Interface/2(trq and spd input request) -> T & w input requested/1
  HTC for parallel HEV and Interface/4(sensors) -> [htcSensors]
  HTC for parallel HEV and Interface/1(requested output) -> [htcReqOut]

== system bd_par_auto2/motor/controller <mc> ==
  note: MOTOR/ CONTROLLER
      | Interface
  trq and spd out requested : Inport  Port=1  LatchInput=off
  electric power in achieved : Inport  Port=2  LatchInput=off
  motor model & interface : Subsystem
      settings: RTWFcnNameOpts=Auto  RTWFileNameOpts=Auto
  electric power in  requested : Outport  Port=1
  "trq and spd out achieved " : Outport  Port=2
  tag scope: mcReqOut=global, mcSensors=global
  wires:
  motor model & interface/3("trq and spd out achieved ") -> "trq and spd out achieved "/1
  electric power in achieved/1 -> motor model & interface/2(electric power in achieved)
  trq and spd out requested/1 -> motor model & interface/1(trq and spd out requested)
  motor model & interface/2(electric power in  requested) -> electric power in  requested/1
  motor model & interface/1(Out Request) -> [mcReqOut]
  [mcControl] -> motor model & interface/3(control)
  motor model & interface/4(sensors) -> [mcSensors]

== system bd_par_auto2/power bus <pb> ==
  note: Power Bus (PB)
  req'd power output (W) : Inport  Port=1  LatchInput=off
  power available from source one (W) : Inport  Port=2  LatchInput=off
  power available from source two (W) : Inport  Port=3  LatchInput=off
  Block NOTES : Subsystem
      settings: RTWFcnNameOpts=Auto  RTWFileNameOpts=Auto
      mask Display: disp('Block\nNOTES')
  help : Subsystem
      settings: OpenFcn=web(['file:\\\' which('fuel_converter.htm')]);  RTWFcnNameOpts=Auto  RTWFileNameOpts=Auto
      mask Display: image(imread('doc_man.jpg'))
  power bus : Subsystem
      settings: RTWFcnNameOpts=Auto  RTWFileNameOpts=Auto
  power req'd from source one (W) : Outport  Port=1
  power req'd from source two (W) : Outport  Port=2
  output power  available at bus : Outport  Port=3
  tag scope: pbReqOut=global, pbSensors=global
  wires:
  power bus/5(sensors) -> [pbSensors]
  power bus/4(power out available) -> output power  available at bus/1
  power bus/3(power in req from  source two) -> power req'd from source two (W)/1
  power bus/2(power in req from  source one) -> power req'd from source one (W)/1
  power bus/1(required out) -> [pbReqOut]
  [pbControl] -> power bus/4(control)
  power available from source two (W)/1 -> power bus/3(power available from source two)
  power available from source one (W)/1 -> power bus/2(power available from source one)
  req'd power output (W)/1 -> power bus/1(power out req)

== system bd_par_auto2/torque coupler <tc> ==
  note: Torque Coupler
  "torque and speed req'd at output side of torque coupler (Nm), (rad/s)" : Inport  Port=1  LatchInput=off
  "torque and speed avail. at main input (Nm), (rad/s)" : Inport  Port=2  LatchInput=off
  "torque and speed avail. at motor input to tc (Nm), (rad/s)" : Inport  Port=3  LatchInput=off
  tc model & interface : Subsystem
      settings: RTWFcnNameOpts=Auto  RTWFileNameOpts=Auto
  "torque and speed req'd at main input to torque coupler (Nm), (rad/s)" : Outport  Port=1  InitialOutput=0
  "torque and speed req'd at motor input to torque coupler (Nm), (rad/s)" : Outport  Port=2  InitialOutput=0
  "torque and speed avail. at output side of torque coupler (Nm), (rad/s)" : Outport  Port=3  InitialOutput=0
  tag scope: tcReqOut=global, tcSensors=global
  wires:
  tc model & interface/5(sensors) -> [tcSensors]
  tc model & interface/4(trq and spd avail. at output side of torque coupler) -> "torque and speed avail. at output side of torque coupler (Nm), (rad/s)"/1
  tc model & interface/3(trq and spd req'd at motor input to torque coupler) -> "torque and speed req'd at motor input to torque coupler (Nm), (rad/s)"/1
  tc model & interface/2(trq and spd req'd at main input) -> "torque and speed req'd at main input to torque coupler (Nm), (rad/s)"/1
  tc model & interface/1(requested output) -> [tcReqOut]
  [tcControl] -> tc model & interface/4(controls)
  "torque and speed avail. at motor input to tc (Nm), (rad/s)"/1 -> tc model & interface/3(trq and spd avail. at motor input to tc)
  "torque and speed avail. at main input (Nm), (rad/s)"/1 -> tc model & interface/2(trq and spd avail. at main input)
  "torque and speed req'd at output side of torque coupler (Nm), (rad/s)"/1 -> tc model & interface/1(trq and spd output request)

== system bd_par_auto2/torque modification  strategy <cs> ==
  note: Torque Modification Strategy
  "original torque and speed req'd (Nm), (rad/s)" : Inport  Port=1  LatchInput=off
  Block NOTES : Subsystem
      settings: RTWFcnNameOpts=Auto  RTWFileNameOpts=Auto
      mask Display: disp('Block\nNOTES')
  help1 : Subsystem
      settings: OpenFcn=web(['file:\\\' which('cs_tips.htm')]);  RTWFcnNameOpts=Auto  RTWFileNameOpts=Auto
      mask Display: image(imread('doc_man.jpg'))
  torque mod  model & interface : Subsystem
      settings: RTWFcnNameOpts=Auto  RTWFileNameOpts=Auto
  "modified torque and speed req'd (Nm), (rad/s)" : Outport  Port=1  InitialOutput=0
  tag scope: tmReqOut=global, tmSensors=global
  wires:
  torque mod  model & interface/3(sensors) -> [tmSensors]
  [tmControl] -> torque mod  model & interface/2(controls)
  "original torque and speed req'd (Nm), (rad/s)"/1 -> torque mod  model & interface/1(trq and spd output request)
  torque mod  model & interface/2(trq and spd input request) -> "modified torque and speed req'd (Nm), (rad/s)"/1
  torque mod  model & interface/1(requested output) -> [tmReqOut]

== system bd_par_auto2/vehicle, wheel, & axle front/rear <wh> 2 axle --> 1 driveline ==
  note: Vehicle, Wheel, and Axle
      | 2 axles --> 1 driveline
  veh spd r : Inport  Port=1  LatchInput=off
  trq & spd a : Inport  Port=2  LatchInput=off
  models and interface : Subsystem  AncestorBlock=|
      | lib_wheel2/vehicle, wheel, & axle
      | front//rear <wh>
      | 2 axle --> 1 driveline/models and interface
      settings: RTWFcnNameOpts=Auto  RTWFileNameOpts=Auto
  trq & spd r : Outport  Port=1  InitialOutput=0
  tag scope: vehReqOut=global, vehSensors=global
  wires:
  veh spd r/1 -> models and interface/1(vehicle speed req'd at end of time step (m/s))
  trq & spd a/1 -> models and interface/2("torque and speed available from drivetrain into axles (Nm), (rad/s)")
  [vehControl] -> models and interface/3(control)
  models and interface/1(requested out) -> [vehReqOut]
  models and interface/2(torque and speed req'd from drivetrain into axles (Nm),(rad/s)) -> trq & spd r/1
  models and interface/3(sensors) -> [vehSensors]
